simulink model "Pacemaker_AOOR2"  (R2020a)
settings: Solver=FixedStepAuto  StartTime=0.0  StopTime=10.0  FixedStep=1e-3  RelTol=1e-3  EnableMultiTasking=on
libraries: etargetslib x17, frdmk64flib x7, simulink x1
settings Model: ExtModeTrigDuration=5  Creator=Tim_G  LastModifiedBy=Panda
settings OptimizationCC: EnhancedBackFolding=on  PassReuseOutputArgsAs=Individual arguments  ZeroExternalMemoryAtStartup=off  ZeroInternalMemoryAtStartup=off  MaxStackSize=64  OptimizeBlockOrder=speed  DifferentSizesBufferReuse=on  OptimizationCustomize=off  EfficientTunableParamExpr=on
settings DebuggingCC: ParameterTunabilityLossMsg=error
settings HardwareCC: ProdBitPerPointer=32  ProdBitPerSizeT=32  ProdBitPerPtrDiffT=32  ProdLargestAtomicInteger=Long  ProdLargestAtomicFloat=Double  ProdEndianess=BigEndian  ProdWordSize=32  ProdHWDeviceType=ARM Compatible->ARM Cortex
settings SFSimCC: MATLABDynamicMemAlloc=off
settings RTWCC: SystemTargetFile=ert.tlc  HardwareBoard=NXP FRDM-K64F  TemplateMakefile=ert_default_tmf  Toolchain=GNU Tools for ARM Embedded Processors
settings CodeAppCC: ForceParamTrailComments=on  IgnoreCustomStorageClasses=off  OperatorAnnotations=on  SimulinkDataObjDesc=on  SFDataObjDesc=on  InsertBlockDesc=on

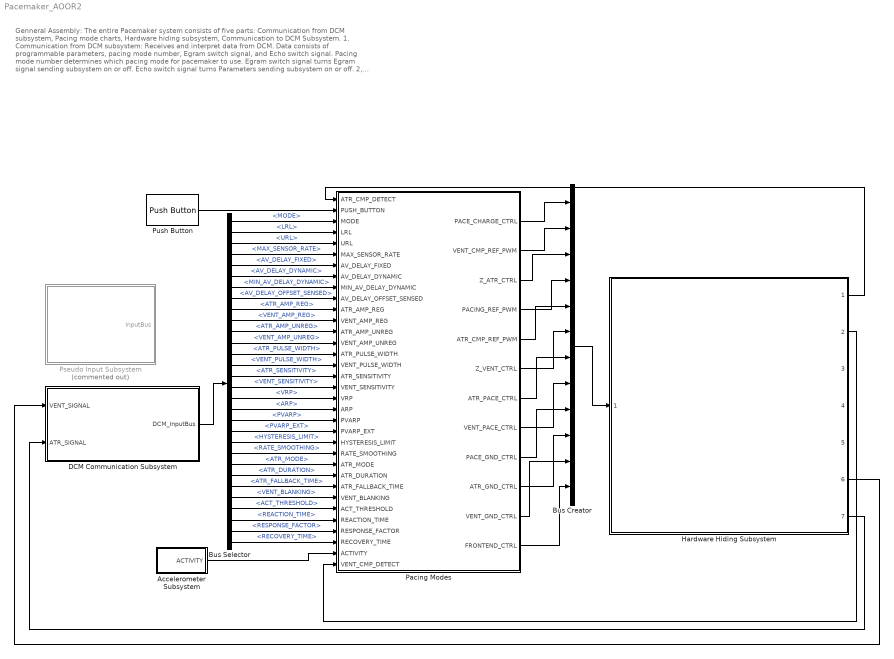
== system Pacemaker_AOOR2 ==
  note: Genneral Assembly:
      |  The entire Pacemaker system consists of five parts: Communication from DCM subsystem, Pacing mode charts, Hardware hiding subsystem, Communication to DCM Subsystem.
      | 1. Communication from DCM subsystem:
      |       Receives and interpret data from DCM. Data consists of programmable parameters, pacing mode number, Egram switch signal, and Echo switch signal.
      |       Pacing mode number determines which pacing mode for pacemaker to use.
      |       Egram switch signal turns Egram signal sending subsystem on or off.
      |       Echo switch signal turns Parameters sending subsystem on or off.
      | 2, Pacing Modes subsystem:
      |       Implementation of different pacing methods. A multiport switch chooses from which pacing mode to output control signals.
      | 3. Hardware hiding subsystem:
      |       Takes control signals as inputs and sends them to the hardware. Also outputs signals received from the hardware.
      | 4. Communication to DCM Subsystem:
      | 	Sends programmable parameters and/or egram signals to DCM if enable signals (ECHO and/or EGRAM) are turned on.
  Accelerometer Subsystem : Subsystem
  Bus Creator : BusCreator  Inputs=12
  Bus Selector : BusSelector  OutputSignals=MODE,LRL,URL,MAX_SENSOR_RATE,AV_DELAY_FIXED,AV_DELAY_DYNAMIC,MIN_AV_DELAY_DYNAMIC,AV_DELAY_OFFSET_SENSED,ATR_AMP_REG,VENT_AMP_REG,ATR_AMP_UNREG,VENT_AMP_UNREG,ATR_PULSE_WIDTH,VENT_PULSE_WIDTH,ATR_SENSITIVITY,VENT_SENSITIVITY,VRP,ARP,PVARP,PVARP_EXT,HYSTERESIS_LIMIT,RATE_SMOOTHING,ATR_MODE,ATR_DURATION,ATR_FALLBACK_TIME,VENT_BLANKING,ACT_THRESHOLD,REACTION_TIME,RESPONSE_FACTOR,RECOVERY_TIME
  DCM Communication Subsystem : Subsystem
  Hardware Hiding Subsystem : Subsystem  ReferencedSubsystem=k64f_hardware_subsystem
  Pacing Modes : Stateflow chart  TreatAsAtomicUnit=on
  Pseudo Input Subsystem : Subsystem  Commented=on
  Push Button : frdmk64flib/Push Button  Whichswitch=SW2  SampleTime1=-1
  wires:
  Hardware Hiding Subsystem/7 -> DCM Communication Subsystem/2(ATR_SIGNAL)
  Hardware Hiding Subsystem/6 -> DCM Communication Subsystem/1(VENT_SIGNAL)
  Push Button/1 -> Pacing Modes/2(PUSH_BUTTON)
  Hardware Hiding Subsystem/1 -> Pacing Modes/1(ATR_CMP_DETECT)
  DCM Communication Subsystem/1(DCM_InputBus) -> Bus Selector/1
  Pacing Modes/1(PACE_CHARGE_CTRL) -> Bus Creator/1
  Pacing Modes/2(VENT_CMP_REF_PWM) -> Bus Creator/2
  Pacing Modes/3(Z_ATR_CTRL) -> Bus Creator/3
  Pacing Modes/4(PACING_REF_PWM) -> Bus Creator/4
  Pacing Modes/5(ATR_CMP_REF_PWM) -> Bus Creator/5
  Pacing Modes/6(Z_VENT_CTRL) -> Bus Creator/6
  Pacing Modes/7(ATR_PACE_CTRL) -> Bus Creator/7
  Pacing Modes/8(VENT_PACE_CTRL) -> Bus Creator/8
  Pacing Modes/9(PACE_GND_CTRL) -> Bus Creator/9
  Pacing Modes/10(ATR_GND_CTRL) -> Bus Creator/10
  Pacing Modes/11(VENT_GND_CTRL) -> Bus Creator/11
  Pacing Modes/12(FRONTEND_CTRL) -> Bus Creator/12
  Bus Creator/1 -> Hardware Hiding Subsystem/1
  Bus Selector/1 -> Pacing Modes/3(MODE)  "<MODE>"
  Bus Selector/2 -> Pacing Modes/4(LRL)  "<LRL>"
  Bus Selector/3 -> Pacing Modes/5(URL)  "<URL>"
  Bus Selector/4 -> Pacing Modes/6(MAX_SENSOR_RATE)  "<MAX_SENSOR_RATE>"
  Bus Selector/5 -> Pacing Modes/7(AV_DELAY_FIXED)  "<AV_DELAY_FIXED>"
  Bus Selector/6 -> Pacing Modes/8(AV_DELAY_DYNAMIC)  "<AV_DELAY_DYNAMIC>"
  Bus Selector/7 -> Pacing Modes/9(MIN_AV_DELAY_DYNAMIC)  "<MIN_AV_DELAY_DYNAMIC>"
  Bus Selector/8 -> Pacing Modes/10(AV_DELAY_OFFSET_SENSED)  "<AV_DELAY_OFFSET_SENSED>"
  Bus Selector/9 -> Pacing Modes/11(ATR_AMP_REG)  "<ATR_AMP_REG>"
  Bus Selector/10 -> Pacing Modes/12(VENT_AMP_REG)  "<VENT_AMP_REG>"
  Bus Selector/11 -> Pacing Modes/13(ATR_AMP_UNREG)  "<ATR_AMP_UNREG>"
  Bus Selector/12 -> Pacing Modes/14(VENT_AMP_UNREG)  "<VENT_AMP_UNREG>"
  Bus Selector/13 -> Pacing Modes/15(ATR_PULSE_WIDTH)  "<ATR_PULSE_WIDTH>"
  Bus Selector/14 -> Pacing Modes/16(VENT_PULSE_WIDTH)  "<VENT_PULSE_WIDTH>"
  Bus Selector/15 -> Pacing Modes/17(ATR_SENSITIVITY)  "<ATR_SENSITIVITY>"
  Bus Selector/16 -> Pacing Modes/18(VENT_SENSITIVITY)  "<VENT_SENSITIVITY>"
  Bus Selector/17 -> Pacing Modes/19(VRP)  "<VRP>"
  Bus Selector/18 -> Pacing Modes/20(ARP)  "<ARP>"
  Bus Selector/19 -> Pacing Modes/21(PVARP)  "<PVARP>"
  Bus Selector/20 -> Pacing Modes/22(PVARP_EXT)  "<PVARP_EXT>"
  Bus Selector/21 -> Pacing Modes/23(HYSTERESIS_LIMIT)  "<HYSTERESIS_LIMIT>"
  Bus Selector/22 -> Pacing Modes/24(RATE_SMOOTHING)  "<RATE_SMOOTHING>"
  Bus Selector/23 -> Pacing Modes/25(ATR_MODE)  "<ATR_MODE>"
  Bus Selector/24 -> Pacing Modes/26(ATR_DURATION)  "<ATR_DURATION>"
  Bus Selector/25 -> Pacing Modes/27(ATR_FALLBACK_TIME)  "<ATR_FALLBACK_TIME>"
  Bus Selector/26 -> Pacing Modes/28(VENT_BLANKING)  "<VENT_BLANKING>"
  Bus Selector/27 -> Pacing Modes/29(ACT_THRESHOLD)  "<ACT_THRESHOLD>"
  Bus Selector/28 -> Pacing Modes/30(REACTION_TIME)  "<REACTION_TIME>"
  Bus Selector/29 -> Pacing Modes/31(RESPONSE_FACTOR)  "<RESPONSE_FACTOR>"
  Bus Selector/30 -> Pacing Modes/32(RECOVERY_TIME)  "<RECOVERY_TIME>"
  Accelerometer Subsystem/1(ACTIVITY) -> Pacing Modes/33(ACTIVITY)
  Hardware Hiding Subsystem/2 -> Pacing Modes/34(VENT_CMP_DETECT)

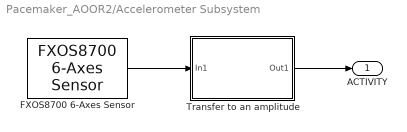
== system Pacemaker_AOOR2/Accelerometer Subsystem ==
  FXOS8700 6-Axes Sensor : frdmk64flib/FXOS8700 6-Axes Sensor  Activesensor=Accelerometer only  ODR=800Hz  HybridODR=400Hz  Accelfullrange=-2g to +2g  SampleTime=-1
  Transfer to an amplitude : Subsystem
  ACTIVITY : Outport
  wires:
  FXOS8700 6-Axes Sensor/1 -> Transfer to an amplitude/1(In1)
  Transfer to an amplitude/1(Out1) -> ACTIVITY/1

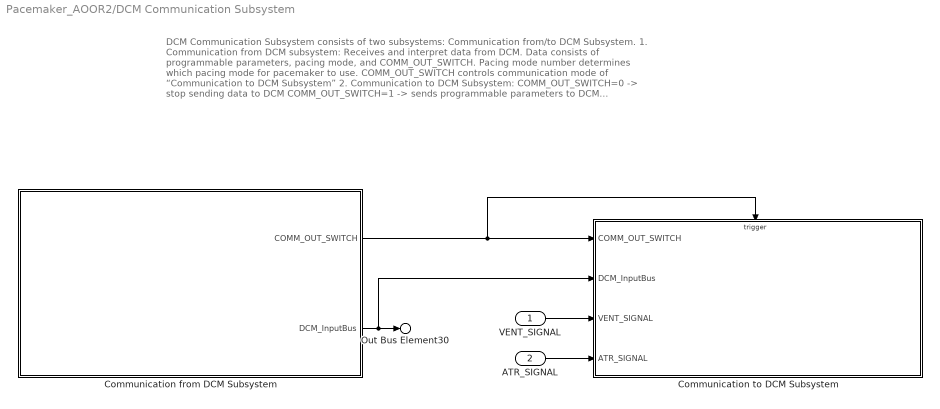
== system Pacemaker_AOOR2/DCM Communication Subsystem ==
  note: DCM Communication Subsystem consists of two subsystems: Communication from/to DCM Subsystem.
      | 1. Communication from DCM subsystem:
      | Receives and interpret data from DCM.
      | Data consists of programmable parameters, pacing mode, and COMM_OUT_SWITCH.
      | Pacing mode number determines which pacing mode for pacemaker to use.
      | COMM_OUT_SWITCH controls communication mode of “Communication to DCM Subsystem”
      | 2. Communication to DCM Subsystem:
      | COMM_OUT_SWITCH=0 -> stop sending data to DCM
      | COMM_OUT_SWITCH=1 -> sends programmable parameters to DCM
      | COMM_OUT_SWITCH=2 -> s ends egram signals to DCM
  VENT_SIGNAL : Inport  OutDataTypeStr=double
  ATR_SIGNAL : Inport  Port=2  OutDataTypeStr=double
  Communication from DCM Subsystem : Subsystem
  Communication to DCM Subsystem : Subsystem  TreatAsAtomicUnit=on
  Out Bus Element30 : Outport  PortName=DCM_InputBus
  wires:
  VENT_SIGNAL/1 -> Communication to DCM Subsystem/3(VENT_SIGNAL)
  ATR_SIGNAL/1 -> Communication to DCM Subsystem/4(ATR_SIGNAL)
  Communication from DCM Subsystem/2(DCM_InputBus) -> Communication to DCM Subsystem/2(DCM_InputBus), Out Bus Element30/1
  Communication from DCM Subsystem/1(COMM_OUT_SWITCH) -> Communication to DCM Subsystem/Trigger, Communication to DCM Subsystem/1(COMM_OUT_SWITCH)

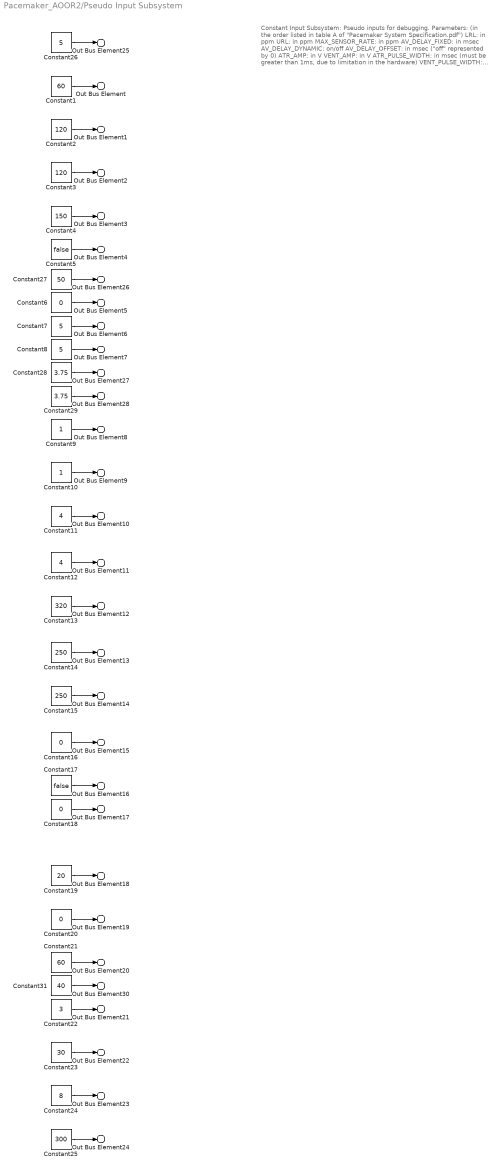
== system Pacemaker_AOOR2/Pseudo Input Subsystem ==
  note: Constant Input Subsystem:
      | Pseudo inputs for debugging.
      |
      | Parameters:
      | (in the order listed in table A of "Pacemaker System Specification.pdf")
      | LRL: in ppm
      | URL: in ppm
      | MAX_SENSOR_RATE: in ppm
      | AV_DELAY_FIXED: in msec
      | AV_DELAY_DYNAMIC: on/off
      | AV_DELAY_OFFSET: in msec ("off" represented by 0)
      | ATR_AMP: in V
      | VENT_AMP: in V
      | ATR_PULSE_WIDTH: in msec (must be greater than 1ms, due to
      | limitation in the hardware)
      | VENT_PULSE_WIDTH: in msec
      | ATR_SENSITIVITY: in V
      | VENT_SENSITIVITY: in V
      | VRP: in msec
      | ARP: in msec
      | PVARP: in msec
      | PVARP_EXT: in msec ("off" represented by 0)
      | HYSTERESIS: off/same choices as LRL (represented by "on")
      | RATE_SMOOTHING: off represented by 0
      | ATR_DURATION: in cardiac cycles
      | ATR_FALLBACK_MODE
      | ATR_FALLBACK_TIME: in sec
      | ACT_THRESHOLD:
      | 0-V-Low
      | 1-Low
      | 2-Med-Low
      | 3-Med
      | 4-Med-High
      | 5-High
      | 6-V-High
      | REACTION_TIME: in sec
      | RESPONSE_FACTOR
      | RECOVERY_TIME: in sec
  Constant1 : Constant  Value=60
  Constant10 : Constant
  Constant11 : Constant  Value=4
  Constant12 : Constant  Value=4
  Constant13 : Constant  Value=320
  Constant14 : Constant  Value=250
  Constant15 : Constant  Value=250
  Constant{6,16,18,20} (4 alike) : Constant  Value=0
  Constant17 : Constant  Value=false
  Constant19 : Constant  Value=20
  Constant2 : Constant  Value=120
  Constant21 : Constant  Value=60
  Constant22 : Constant  Value=3
  Constant23 : Constant  Value=30
  Constant24 : Constant  Value=8
  Constant25 : Constant  Value=300
  Constant26 : Constant  Value=5
  Constant27 : Constant  Value=50
  Constant28 : Constant  Value=3.75
  Constant29 : Constant  Value=3.75
  Constant3 : Constant  Value=120
  Constant31 : Constant  Value=40
  Constant4 : Constant  Value=150
  Constant5 : Constant  Value=false
  Constant7 : Constant  Value=5
  Constant8 : Constant  Value=5
  Constant9 : Constant
  Out Bus Element : Outport  PortName=InputBus  Element=LRL
  Out Bus Element1 : Outport  PortName=InputBus  Element=URL
  Out Bus Element2 : Outport  PortName=InputBus  Element=MAX_SENSOR_RATE
  Out Bus Element3 : Outport  PortName=InputBus  Element=AV_DELAY_FIXED
  Out Bus Element4 : Outport  PortName=InputBus  Element=AV_DELAY_DYNAMIC
  Out Bus Element5 : Outport  PortName=InputBus  Element=AV_DELAY_OFFSET_SENSED
  Out Bus Element6 : Outport  PortName=InputBus  Element=ATR_AMP_REG
  Out Bus Element7 : Outport  PortName=InputBus  Element=VENT_AMP_REG
  Out Bus Element8 : Outport  PortName=InputBus  Element=ATR_PULSE_WIDTH
  Out Bus Element9 : Outport  PortName=InputBus  Element=VENT_PULSE_WIDTH
  Out Bus Element10 : Outport  PortName=InputBus  Element=ATR_SENSITIVITY
  Out Bus Element11 : Outport  PortName=InputBus  Element=VENT_SENSITIVITY
  Out Bus Element12 : Outport  PortName=InputBus  Element=VRP
  Out Bus Element13 : Outport  PortName=InputBus  Element=ARP
  Out Bus Element14 : Outport  PortName=InputBus  Element=PVARP
  Out Bus Element15 : Outport  PortName=InputBus  Element=PVARP_EXT
  Out Bus Element16 : Outport  PortName=InputBus  Element=HYSTERESIS
  Out Bus Element17 : Outport  PortName=InputBus  Element=RATE_SMOOTHING
  Out Bus Element18 : Outport  PortName=InputBus  Element=ATR_DURATION
  Out Bus Element19 : Outport  PortName=InputBus  Element=ATR_FALLBACK_MODE
  Out Bus Element20 : Outport  PortName=InputBus  Element=ATR_FALLBACK_TIME
  Out Bus Element21 : Outport  PortName=InputBus  Element=ACT_THRESHOLD
  Out Bus Element22 : Outport  PortName=InputBus  Element=REACTION_TIME
  Out Bus Element23 : Outport  PortName=InputBus  Element=RESPONSE_FACTOR
  Out Bus Element24 : Outport  PortName=InputBus  Element=RECOVERY_TIME
  Out Bus Element25 : Outport  PortName=InputBus  Element=MODE
  Out Bus Element26 : Outport  PortName=InputBus  Element=MIN_AV_DELAY_DYNAMIC
  Out Bus Element27 : Outport  PortName=InputBus  Element=ATR_AMP_UNREG
  Out Bus Element28 : Outport  PortName=InputBus  Element=VENT_AMP_UNREG
  Out Bus Element30 : Outport  PortName=InputBus  Element=VENT_BLANKING
  wires:
  Constant1/1 -> Out Bus Element/1
  Constant2/1 -> Out Bus Element1/1
  Constant4/1 -> Out Bus Element3/1
  Constant3/1 -> Out Bus Element2/1
  Constant5/1 -> Out Bus Element4/1
  Constant6/1 -> Out Bus Element5/1
  Constant8/1 -> Out Bus Element7/1
  Constant7/1 -> Out Bus Element6/1
  Constant10/1 -> Out Bus Element9/1
  Constant11/1 -> Out Bus Element10/1
  Constant9/1 -> Out Bus Element8/1
  Constant13/1 -> Out Bus Element12/1
  Constant12/1 -> Out Bus Element11/1
  Constant14/1 -> Out Bus Element13/1
  Constant15/1 -> Out Bus Element14/1
  Constant19/1 -> Out Bus Element18/1
  Constant18/1 -> Out Bus Element17/1
  Constant16/1 -> Out Bus Element15/1
  Constant17/1 -> Out Bus Element16/1
  Constant25/1 -> Out Bus Element24/1
  Constant24/1 -> Out Bus Element23/1
  Constant23/1 -> Out Bus Element22/1
  Constant22/1 -> Out Bus Element21/1
  Constant20/1 -> Out Bus Element19/1
  Constant21/1 -> Out Bus Element20/1
  Constant26/1 -> Out Bus Element25/1
  Constant27/1 -> Out Bus Element26/1
  Constant28/1 -> Out Bus Element27/1
  Constant29/1 -> Out Bus Element28/1
  Constant31/1 -> Out Bus Element30/1

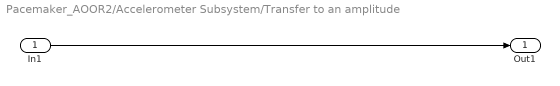
== system Pacemaker_AOOR2/Accelerometer Subsystem/Transfer to an amplitude ==
  In1 : Inport
  Out1 : Outport
  wires:
  In1/1 -> Out1/1

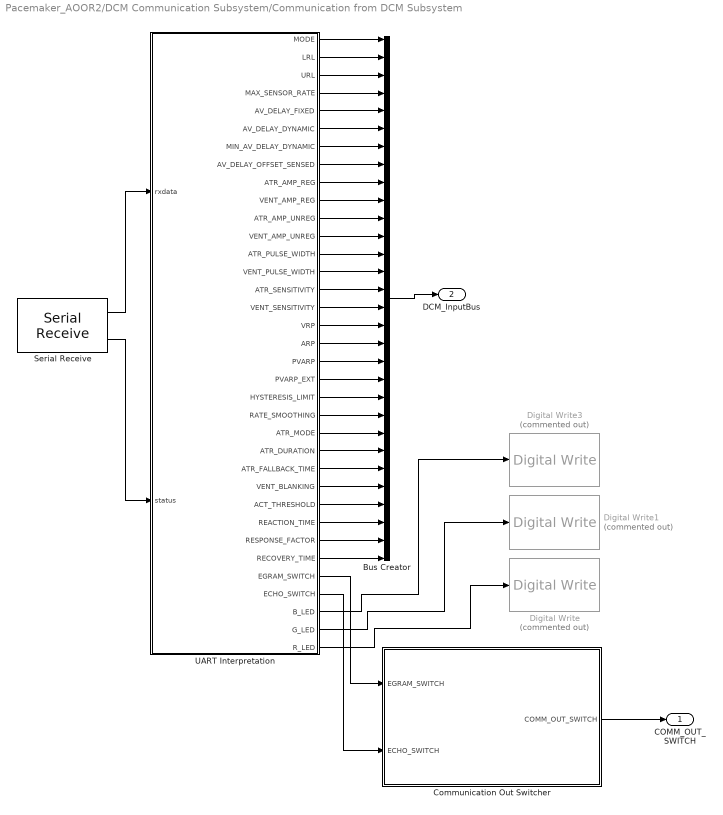
== system Pacemaker_AOOR2/DCM Communication Subsystem/Communication from DCM Subsystem ==
  Bus Creator : BusCreator  Inputs=30
  Communication Out Switcher : Stateflow chart  TreatAsAtomicUnit=on
  Digital Write : frdmk64flib/Digital Write  Commented=on  Whichpin=RED_LED
  Digital Write1 : frdmk64flib/Digital Write  Commented=on  Whichpin=GREEN_LED
  Digital Write3 : frdmk64flib/Digital Write  Commented=on  Whichpin=BLUE_LED
  Serial Receive : frdmk64flib/Serial Receive  SCIModule=0  Baudrate=uint32(9600)  Parity=None  StopBits=1  HardwareFlowControl=None  ByteOrder=LittleEndian  DataType=uint8  DataLength=59  BlockingMode=off  OutputStatus=on  SampleTime=-1
  UART Interpretation : Stateflow chart  TreatAsAtomicUnit=on
  COMM_OUT_SWITCH : Outport
  DCM_InputBus : Outport  Port=2
  wires:
  UART Interpretation/5(AV_DELAY_FIXED) -> Bus Creator/5
  UART Interpretation/14(VENT_PULSE_WIDTH) -> Bus Creator/14
  UART Interpretation/10(VENT_AMP_REG) -> Bus Creator/10
  UART Interpretation/17(VRP) -> Bus Creator/17
  UART Interpretation/6(AV_DELAY_DYNAMIC) -> Bus Creator/6
  UART Interpretation/9(ATR_AMP_REG) -> Bus Creator/9
  UART Interpretation/27(ACT_THRESHOLD) -> Bus Creator/27
  UART Interpretation/24(ATR_DURATION) -> Bus Creator/24
  UART Interpretation/18(ARP) -> Bus Creator/18
  UART Interpretation/8(AV_DELAY_OFFSET_SENSED) -> Bus Creator/8
  UART Interpretation/7(MIN_AV_DELAY_DYNAMIC) -> Bus Creator/7
  Serial Receive/2 -> UART Interpretation/2(status)
  UART Interpretation/3(URL) -> Bus Creator/3
  UART Interpretation/26(VENT_BLANKING) -> Bus Creator/26
  UART Interpretation/13(ATR_PULSE_WIDTH) -> Bus Creator/13
  UART Interpretation/15(ATR_SENSITIVITY) -> Bus Creator/15
  UART Interpretation/11(ATR_AMP_UNREG) -> Bus Creator/11
  UART Interpretation/16(VENT_SENSITIVITY) -> Bus Creator/16
  UART Interpretation/30(RECOVERY_TIME) -> Bus Creator/30
  UART Interpretation/20(PVARP_EXT) -> Bus Creator/20
  UART Interpretation/29(RESPONSE_FACTOR) -> Bus Creator/29
  UART Interpretation/19(PVARP) -> Bus Creator/19
  Serial Receive/1 -> UART Interpretation/1(rxdata)
  UART Interpretation/4(MAX_SENSOR_RATE) -> Bus Creator/4
  UART Interpretation/23(ATR_MODE) -> Bus Creator/23
  UART Interpretation/22(RATE_SMOOTHING) -> Bus Creator/22
  UART Interpretation/12(VENT_AMP_UNREG) -> Bus Creator/12
  UART Interpretation/28(REACTION_TIME) -> Bus Creator/28
  UART Interpretation/25(ATR_FALLBACK_TIME) -> Bus Creator/25
  UART Interpretation/21(HYSTERESIS_LIMIT) -> Bus Creator/21
  UART Interpretation/2(LRL) -> Bus Creator/2
  UART Interpretation/1(MODE) -> Bus Creator/1
  Bus Creator/1 -> DCM_InputBus/1
  Communication Out Switcher/1(COMM_OUT_SWITCH) -> COMM_OUT_SWITCH/1
  UART Interpretation/31(EGRAM_SWITCH) -> Communication Out Switcher/1(EGRAM_SWITCH)
  UART Interpretation/32(ECHO_SWITCH) -> Communication Out Switcher/2(ECHO_SWITCH)
  UART Interpretation/35(R_LED) -> Digital Write/1
  UART Interpretation/33(B_LED) -> Digital Write3/1
  UART Interpretation/34(G_LED) -> Digital Write1/1

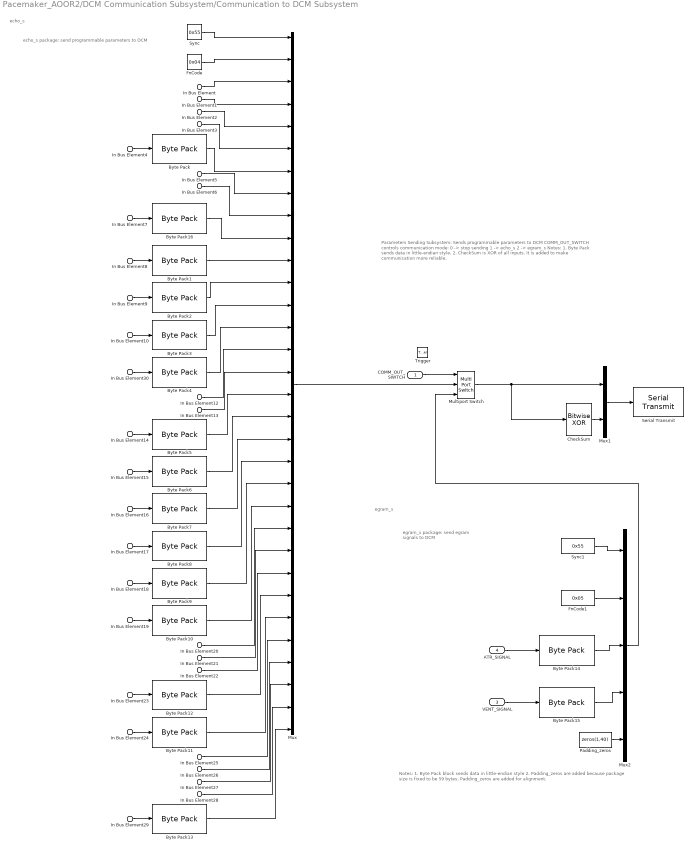
== system Pacemaker_AOOR2/DCM Communication Subsystem/Communication to DCM Subsystem ==
  note: egram_s package:
      | send egram signals to DCM
  note: echo_s package:
      | send programmable parameters to DCM
  note: echo_s
  note: egram_s
  note: Parameters Sending Subsystem:
      | Sends programmable parameters to DCM
      | COMM_OUT_SWITCH controls communication mode:
      | 0 -> stop sending
      | 1 -> echo_s
      | 2 -> egram_s
      | Notes:
      | 1. Byte Pack sends data in little-endian style.
      | 2. CheckSum is XOR of all inputs. It is added to make communication more reliable.
  note: Notes:
      | 1. Byte Pack block sends data in little-endian style
      | 2. Padding_zeros are added because package size is fixed to be 59 bytes. Padding_zeros are added for alignment.
  COMM_OUT_SWITCH : Inport
  In Bus Element : Inport  Port=2  PortName=DCM_InputBus  Element=MODE
  In Bus Element1 : Inport  Port=2  PortName=DCM_InputBus  Element=LRL
  In Bus Element2 : Inport  Port=2  PortName=DCM_InputBus  Element=URL
  In Bus Element3 : Inport  Port=2  PortName=DCM_InputBus  Element=MAX_SENSOR_RATE
  In Bus Element4 : Inport  Port=2  PortName=DCM_InputBus  Element=AV_DELAY_FIXED
  In Bus Element5 : Inport  Port=2  PortName=DCM_InputBus  Element=AV_DELAY_DYNAMIC
  In Bus Element6 : Inport  Port=2  PortName=DCM_InputBus  Element=MIN_AV_DELAY_DYNAMIC
  In Bus Element7 : Inport  Port=2  PortName=DCM_InputBus  Element=AV_DELAY_OFFSET_SENSED
  In Bus Element8 : Inport  Port=2  PortName=DCM_InputBus  Element=ATR_AMP_REG
  In Bus Element9 : Inport  Port=2  PortName=DCM_InputBus  Element=VENT_AMP_REG
  In Bus Element10 : Inport  Port=2  PortName=DCM_InputBus  Element=ATR_AMP_UNREG
  In Bus Element12 : Inport  Port=2  PortName=DCM_InputBus  Element=ATR_PULSE_WIDTH
  In Bus Element13 : Inport  Port=2  PortName=DCM_InputBus  Element=VENT_PULSE_WIDTH
  In Bus Element14 : Inport  Port=2  PortName=DCM_InputBus  Element=ATR_SENSITIVITY
  In Bus Element15 : Inport  Port=2  PortName=DCM_InputBus  Element=VENT_SENSITIVITY
  In Bus Element16 : Inport  Port=2  PortName=DCM_InputBus  Element=VRP
  In Bus Element17 : Inport  Port=2  PortName=DCM_InputBus  Element=ARP
  In Bus Element18 : Inport  Port=2  PortName=DCM_InputBus  Element=PVARP
  In Bus Element19 : Inport  Port=2  PortName=DCM_InputBus  Element=PVARP_EXT
  In Bus Element20 : Inport  Port=2  PortName=DCM_InputBus  Element=HYSTERESIS_LIMIT
  In Bus Element21 : Inport  Port=2  PortName=DCM_InputBus  Element=RATE_SMOOTHING
  In Bus Element22 : Inport  Port=2  PortName=DCM_InputBus  Element=ATR_MODE
  In Bus Element23 : Inport  Port=2  PortName=DCM_InputBus  Element=ATR_DURATION
  In Bus Element24 : Inport  Port=2  PortName=DCM_InputBus  Element=ATR_FALLBACK_TIME
  In Bus Element25 : Inport  Port=2  PortName=DCM_InputBus  Element=VENT_BLANKING
  In Bus Element26 : Inport  Port=2  PortName=DCM_InputBus  Element=ACT_THRESHOLD
  In Bus Element27 : Inport  Port=2  PortName=DCM_InputBus  Element=REACTION_TIME
  In Bus Element28 : Inport  Port=2  PortName=DCM_InputBus  Element=RESPONSE_FACTOR
  In Bus Element29 : Inport  Port=2  PortName=DCM_InputBus  Element=RECOVERY_TIME
  In Bus Element30 : Inport  Port=2  PortName=DCM_InputBus  Element=VENT_AMP_UNREG
  VENT_SIGNAL : Inport  Port=3  OutDataTypeStr=double
  ATR_SIGNAL : Inport  Port=4  OutDataTypeStr=double
  Trigger : TriggerPort  VariantControl=Variant  InitialTriggerSignalState=zero  PortDimensions=1
  Byte Pack{,7..13} (8 alike) : etargetslib/Byte Pack  datatypes={'uint16'}  byteAlign=1
  Byte Pack{1..6} (6 alike) : etargetslib/Byte Pack  datatypes={'single'}  byteAlign=1
  Byte Pack14 : etargetslib/Byte Pack  datatypes={'double'}  byteAlign=1
  Byte Pack15 : etargetslib/Byte Pack  datatypes={'double'}  byteAlign=1
  Byte Pack16 : etargetslib/Byte Pack  datatypes={'int8'}  byteAlign=1
  CheckSum : simulink/Logic and Bit Operations/Bitwise Operator  logicop=XOR  UseBitMask=off  BitMask=bin2dec('11011001')  BitMaskRealWorld=Stored Integer
  FnCode : Constant  Value=0x04  OutDataTypeStr=uint8
  FnCode1 : Constant  Value=0x05  OutDataTypeStr=uint8
  Multiport Switch : MultiPortSwitch  Inputs=2
  Mux : Mux  Inputs=32
  Mux1 : Mux  Inputs=2
  Mux2 : Mux  Inputs=5
  Padding_zeros : Constant  Value=zeros(1,40)  VectorParams1D=off  OutDataTypeStr=uint8
  Serial Transmit : frdmk64flib/Serial Transmit  SCIModule=0  Baudrate=uint32(9600)  Parity=None  StopBits=1  HardwareFlowControl=None  ByteOrder=LittleEndian  BlockingMode=on  OutputStatus=off
  Sync : Constant  Value=0x55  OutDataTypeStr=uint8
  Sync1 : Constant  Value=0x55  OutDataTypeStr=uint8
  wires:
  In Bus Element25/1 -> Mux/28
  Byte Pack13/1 -> Mux/32
  Byte Pack11/1 -> Mux/27
  In Bus Element20/1 -> Mux/23
  Byte Pack12/1 -> Mux/26
  Byte Pack8/1 -> Mux/20
  Byte Pack10/1 -> Mux/22
  In Bus Element/1 -> Mux/3
  Byte Pack9/1 -> Mux/21
  Byte Pack7/1 -> Mux/19
  Byte Pack5/1 -> Mux/17
  In Bus Element12/1 -> Mux/15
  Byte Pack1/1 -> Mux/11
  Byte Pack6/1 -> Mux/18
  In Bus Element6/1 -> Mux/9
  In Bus Element26/1 -> Mux/29
  Byte Pack3/1 -> Mux/13
  Byte Pack2/1 -> Mux/12
  Byte Pack/1 -> Mux/7
  In Bus Element21/1 -> Mux/24
  In Bus Element22/1 -> Mux/25
  In Bus Element28/1 -> Mux/31
  In Bus Element27/1 -> Mux/30
  Byte Pack4/1 -> Mux/14
  In Bus Element13/1 -> Mux/16
  In Bus Element5/1 -> Mux/8
  In Bus Element1/1 -> Mux/4
  In Bus Element4/1 -> Byte Pack/1
  In Bus Element3/1 -> Mux/6
  In Bus Element2/1 -> Mux/5
  FnCode/1 -> Mux/2
  Sync/1 -> Mux/1
  Mux1/1 -> Serial Transmit/1
  CheckSum/1 -> Mux1/2
  Sync1/1 -> Mux2/1
  Mux/1 -> Multiport Switch/2
  Multiport Switch/1 -> CheckSum/1, Mux1/1
  Byte Pack14/1 -> Mux2/3
  Byte Pack15/1 -> Mux2/4
  FnCode1/1 -> Mux2/2
  Mux2/1 -> Multiport Switch/3
  Padding_zeros/1 -> Mux2/5
  Byte Pack16/1 -> Mux/10
  In Bus Element7/1 -> Byte Pack16/1
  In Bus Element8/1 -> Byte Pack1/1
  In Bus Element9/1 -> Byte Pack2/1
  In Bus Element10/1 -> Byte Pack3/1
  In Bus Element30/1 -> Byte Pack4/1
  In Bus Element14/1 -> Byte Pack5/1
  In Bus Element15/1 -> Byte Pack6/1
  In Bus Element16/1 -> Byte Pack7/1
  In Bus Element17/1 -> Byte Pack8/1
  In Bus Element18/1 -> Byte Pack9/1
  In Bus Element19/1 -> Byte Pack10/1
  In Bus Element29/1 -> Byte Pack13/1
  In Bus Element23/1 -> Byte Pack12/1
  In Bus Element24/1 -> Byte Pack11/1
  ATR_SIGNAL/1 -> Byte Pack14/1
  VENT_SIGNAL/1 -> Byte Pack15/1
  COMM_OUT_SWITCH/1 -> Multiport Switch/1

== stateflow chart Pacemaker_AOOR2/DCM Communication Subsystem/Communication from DCM Subsystem/Communication Out Switcher ==
  note: Communication out Switcher:
      | % help switch between echo and egram communication modes
      | 	if ECHO_SWITCH is true:
      | 		send only 1 programmable-parameters package
      | 	If EGRAM_SWITCH is true:
      | 		send a egram data package once per 1ms by switching COMM_OUT_SWITCH between 0/1
  state egram_stop
    % egram low stage
    % wait for 1ms to send next egram package
    entry:
    COMM_OUT_SWITCH=0;
  state comm_stop
    % stop communication
    entry:
    COMM_OUT_SWITCH=0;
  state egram_pulse
    % egram high stage (pulse)
    % send a egram data package
    entry:
    COMM_OUT_SWITCH=2;
  state echo_s_pulse
    % send a programmable-parameters package
    % 1ms delay allows enough time for DCM to read
    entry:
    COMM_OUT_SWITCH=1;
  (default) -> comm_stop
  egram_stop -> comm_stop [order 2] : [ECHO_SWITCH==true]
  comm_stop -> egram_stop [order 2] : [EGRAM_SWITCH==true]
  comm_stop -> (junction 24) [order 1] : [ECHO_SWITCH==true]
  echo_s_pulse -> comm_stop
  egram_pulse -> comm_stop [order 1] : [EGRAM_SWITCH==false | ECHO_SWITCH==true]
  egram_pulse -> egram_stop [order 2]
  egram_stop -> egram_pulse [order 1] : [after(100,msec)]
  (junction 24) -> echo_s_pulse : [after(1,msec)]
  data: EGRAM_SWITCH input boolean; COMM_OUT_SWITCH output uint8; ECHO_SWITCH input boolean

== stateflow chart Pacemaker_AOOR2/DCM Communication Subsystem/Communication from DCM Subsystem/UART Interpretation ==
  settings: executeAtInitialization=1
  state set_r
    entry:
    % store parameters values from DCM
    MODE = data(3);
    LRL = data(4);
    URL = data(5);
    MAX_SENSOR_RATE = data(6);
    AV_DELAY_FIXED = typecast(data(7: 8), 'uint16');
    AV_DELAY_DYNAMIC = data(9);
    MIN_AV_DELAY_DYNAMIC = data(10);
    AV_DELAY_OFFSET_SENSED =  typecast(data(11), 'int8');
    ATR_AMP_REG = typecast(data(12: 15), 'single');
    VENT_AMP_REG = typecast(data(16: 19), 'single');
    ATR_AMP_UNREG = typecast(data(20: 23), 'single');
    VENT_AMP_UNREG = typecast(data(24: 27), 'single');
    ATR_PULSE_WIDTH = data(28);
    VENT_PULSE_WIDTH = data(29);
    ATR_SENSITIVITY = typecast(data(30: 33), 'single');
    VENT_SENSITIVITY = typecast(data(34: 37), 'single');
    VRP = typecast(data(38: 39), 'uint16');
    ARP = typecast(data(40: 41), 'uint16');
    PVARP = typecast(data(42: 43), 'uint16');
    PVARP_EXT = typecast(data(44: 45), 'uint16');
    HYSTERESIS_LIMIT = data(46);
    RATE_SMOOTHING = data(47);
    ATR_MODE = data(48);
    ATR_DURATION = typecast(data(49: 50), 'uint16');
    ATR_FALLBACK_TIME = typecast(data(51: 52), 'uint16');
    VENT_BLANKING = data(53);
    ACT_THRESHOLD = data(54);
    REACTION_TIME = data(55);
    RESPONSE_FACTOR = data(56);
    RECOVERY_TIME = typecast(data(57: 58), 'uint16');
    B_LED=true;
  note: This chart interprets data received from DCM communication.
      | There’re four types of package pacemaker can receive: set_r, echo_r, egram_r, and stopegram_r. (Documentation section 3.3.2)
      | After a package of 59 bytes is received, status==0, then operate the following 4 steps:
      | 1. Validate Sync byte. If not valid, ignore this package and wait for next package.
      | 2. Validate Checksum. If not valid, ignore this package and wait for next package.
      | 3. Operate according to FnCode (set_r, echo_r, egram_r, or stopegram_r).
      | 4. Wait for next package.
      |
      | Note:
      | The matlab function bitsxor() is used to calculate checksum of data received.
  state echo_r
    % send a parameter package to DCM
    entry:
    ECHO_SWITCH=true;
    G_LED=true;
  state Init
    entry:
    % parameters have default values if no data received
    MODE=5; % change to DDD in the future
    LRL=60;
    URL=120;
    MAX_SENSOR_RATE=120;
    AV_DELAY_FIXED=150;
    AV_DELAY_DYNAMIC=0;
    MIN_AV_DELAY_DYNAMIC=50;
    AV_DELAY_OFFSET_SENSED=0;
    ATR_AMP_REG=5;
    VENT_AMP_REG=5;
    ATR_AMP_UNREG=3.75;
    VENT_AMP_UNREG=3.75;
    ATR_PULSE_WIDTH=1;
    VENT_PULSE_WIDTH=1;
    ATR_SENSITIVITY=4;
    VENT_SENSITIVITY=4;
    VRP=320;
    ARP=250;
    PVARP=250;
    PVARP_EXT=0;
    HYSTERESIS_LIMIT=0;
    RATE_SMOOTHING=0;
    ATR_MODE=0;
    ATR_DURATION=20;
    ATR_FALLBACK_TIME=60;
    VENT_BLANKING=40;
    ACT_THRESHOLD=3;
    REACTION_TIME=30;
    RESPONSE_FACTOR=8;
    RECOVERY_TIME=300;
    % local variables that turn egram/echo communication
    % out modules on/off
    EGRAM_SWITCH=false;
    ECHO_SWITCH=false;
  state Checksum
    entry:
    % compare checksum first
    % if checksum is valid, operate according to FnCode
    CHECKSUM=data(59);
    CHECKSUM_REAL=bitsxor(data(1:58));
  state Standby
    %Waiting for Data
    exit:
    % rxdata must be stored initially, otherwise rxdata
    % changes after Checksum. The reason is rxdata
    % reset to zeros after all data have been read
    data=rxdata;
  state stopegram_r
    % stop sending egram to DCM
    entry:
    EGRAM_SWITCH=false;
    R_LED=false;
  state egram_r
    % start sending a egram package
    % to DCM every 1ms
    entry:
    EGRAM_SWITCH=true;
    R_LED=true;
  set_r -> Standby
  (default) -> Init
  (junction 45) -> set_r [order 1] : [data(2)==0x00]
  echo_r -> Standby : {ECHO_SWITCH=false}
  (junction 45) -> Standby [order 5]
  (junction 45) -> echo_r [order 2] : [data(2)==0x01]
  Checksum -> Standby [order 2]
  (junction 41) -> Standby [order 2]
  Checksum -> (junction 45) [order 1] : [CHECKSUM_REAL==CHECKSUM]
  (junction 45) -> egram_r [order 3] : [data(2)==0x02]
  (junction 45) -> stopegram_r [order 4] : [data(2)==0x03]
  Init -> Standby
  Standby -> (junction 41) : [status==0]
  (junction 41) -> Checksum [order 1] : [rxdata(1)==0x55]{B_LED=false;G_LED=false}
  egram_r -> Standby
  stopegram_r -> Standby
  data: checksum function_output uint8 size=1; data_array function_input uint8; MODE output uint8; LRL output uint8; URL output uint8; MAX_SENSOR_RATE output uint8; AV_DELAY_FIXED output uint16; AV_DELAY_DYNAMIC output uint8; MIN_AV_DELAY_DYNAMIC output uint8; AV_DELAY_OFFSET_SENSED output int8; ATR_AMP_REG output single; VENT_AMP_REG output single; ATR_AMP_UNREG output single; VENT_AMP_UNREG output single; ATR_PULSE_WIDTH output uint8; VENT_PULSE_WIDTH output uint8; ATR_SENSITIVITY output single; VENT_SENSITIVITY output single; VRP output uint16; ARP output uint16; PVARP output uint16; PVARP_EXT output uint16; HYSTERESIS_LIMIT output uint8; RATE_SMOOTHING output uint8; ATR_MODE output uint8; ATR_DURATION output uint16; ATR_FALLBACK_TIME output uint16; VENT_BLANKING output uint8; rxdata input uint8; status input uint8; ACT_THRESHOLD output uint8; REACTION_TIME output uint8; RESPONSE_FACTOR output uint8; RECOVERY_TIME output uint16; CHECKSUM_REAL local uint8 size=1; CHECKSUM local uint8 size=1; EGRAM_SWITCH output boolean; ECHO_SWITCH output boolean; B_LED output boolean; data local uint8; G_LED output; R_LED output
  function checksum=bitsxor(data_array):
    | function checksum=bitsxor(data_array)
    |     % calculate checksum
    |     % input: data_array is array of uint8 numbers
    |     % output: checksum (uint8) is bit-wise XOR of all uint8 data in the array
    |     checksum=data_array(1);
    |     for i=2:length(data_array)
    |         checksum = bitxor(checksum,data_array(i)); 
    |     end
    | end

== stateflow chart Pacemaker_AOOR2/Pacing Modes ==
  state Pacing_Modes_Switch
    % switch pacing modes according to MODE
    % similar to switch case in C = C + 1
  state AOO
    note: AOO Pacing Mode:
        |
        | Inputs:
        | ppm=LRL; (1/automatic interval)
        | ATR_AMP_REG; (amplitude in V)
        | ATR_PULSE_WIDTH; (in msec)
    state Init
      entry:
      VENT_CMP_REF_PWM=100;
      ATR_CMP_REF_PWM=100;
      FRONTEND_CTRL=false;
    state Charging
      %% Charge C22
      entry:
      ATR_PACE_CTRL = false;
      VENT_PACE_CTRL = false;
      PACING_REF_PWM = double(ATR_AMP_REG*20);
      % Because 0-100% PWM corresponds to 0-5V output,
      % PWM duty cycle = ATR_AMP_REG/5*100;
      PACE_CHARGE_CTRL = true;
      %% Discharge C21
      PACE_GND_CTRL = true;
      Z_ATR_CTRL = false;
      Z_VENT_CTRL = false;
      ATR_GND_CTRL = true;
      VENT_GND_CTRL = false;
    state Pacing
      entry:
      PACE_CHARGE_CTRL = false;
      PACE_GND_CTRL = true;
      ATR_PACE_CTRL = true;
      ATR_GND_CTRL = false;
      Z_ATR_CTRL = false;
      Z_VENT_CTRL =false;
      VENT_GND_CTRL = false;
      VENT_PACE_CTRL = false;
    (default) -> AOO.Init
    AOO.Charging -> AOO.Pacing : [after(60/LRL,sec)]
    AOO.Init -> AOO.Charging
    AOO.Pacing -> AOO.Charging : [after(ATR_PULSE_WIDTH,msec)]
  state VOO [commented out]
    note: VOO Pacing Mode:
        |
        | Inputs:
        | ppm=LRL; (1/automatic interval)
        | VENT_AMP_REG; (amplitude in V)
        | VENT_PULSE_WIDTH; (in msec)
    state Init [commented out]
      entry:
      VENT_CMP_REF_PWM=100;
      ATR_CMP_REF_PWM=100;
      FRONTEND_CTRL=false;
    state Charging [commented out]
      entry:
      %% Charge C22
      ATR_PACE_CTRL = false;
      VENT_PACE_CTRL = false;
      PACING_REF_PWM = double(VENT_AMP_REG*20);
      % Because 0-100% PWM corresponds to 0-5V output,
      %PWM duty cycle = VENT_AMP_REG/5*100;
      PACE_CHARGE_CTRL = true;
      %% Discharge C21
      PACE_GND_CTRL = true;
      Z_ATR_CTRL = false;
      Z_VENT_CTRL = false;
      ATR_GND_CTRL = false;
      VENT_GND_CTRL = true;
    state Pacing [commented out]
      entry:
      PACE_CHARGE_CTRL = false;
      PACE_GND_CTRL = true;
      ATR_PACE_CTRL = false;
      ATR_GND_CTRL = false;
      Z_ATR_CTRL = false;
      Z_VENT_CTRL = false;
      VENT_GND_CTRL = false;
      VENT_PACE_CTRL = true;
    (default) -> VOO.Init [commented out]
    VOO.Charging -> VOO.Pacing [commented out] : [after(60/LRL,sec)]
    VOO.Pacing -> VOO.Charging [commented out] : [after(VENT_PULSE_WIDTH,msec)]
    VOO.Init -> VOO.Charging [commented out]
  state AAI [commented out]
    state REF_delay [commented out]
    note: Inputs:
        | ATR_SENSITIVITY (sensing threshold in V)
        | ARP; (atrial refactory period, in msec)
        | ppm= LRL; (1/automatic interval)
        | ATR_AMP_REG (amplitude in V)
        | ATR_PULSE_WIDTH; (pulse width in msec)
        | ATR_CMP_DETECT; (sensing signal from hardware)
    state Sensing [commented out]
      entry:
      FRONTEND_CTRL = true;
      VENT_CMP_REF_PWM=100;
      ATR_CMP_REF_PWM = double(ATR_SENSITIVITY*20);
      % see explanation for ...REF_PWM in section 2.3.4 of the Document
    state Charge [commented out]
      entry:
      %% Charge C22
      ATR_PACE_CTRL = false;
      VENT_PACE_CTRL = false;
      PACING_REF_PWM = double(ATR_AMP_REG*20);
      % Because 0-100% PWM corresponds to 0-5V output,
      % PWM duty cycle = ATR_AMP_REG/5*100;
      PACE_CHARGE_CTRL = true;
      %% Discharge C21
      PACE_GND_CTRL = true;
      Z_ATR_CTRL = false;
      Z_VENT_CTRL = false;
      ATR_GND_CTRL = true;
      VENT_GND_CTRL = false;
    state Pacing [commented out]
      entry:
      PACE_CHARGE_CTRL = false;
      PACE_GND_CTRL = true;
      ATR_PACE_CTRL = true;
      ATR_GND_CTRL = false;
      Z_ATR_CTRL = false;
      Z_VENT_CTRL = false;
      VENT_GND_CTRL = false;
      VENT_PACE_CTRL = false;
    AAI.REF_delay -> AAI.Pacing [commented out] : [after(60000/LRL - double(ATR_PULSE_WIDTH) - double(ARP), msec)]
    Charge -> AAI.REF_delay [commented out] : [after(ARP,msec)]
    AAI.REF_delay -> Charge [commented out] : [ATR_CMP_DETECT == true || PUSH_BUTTON==true]
    (default) -> Sensing [commented out]
    Sensing -> Charge [commented out]
    AAI.Pacing -> Charge [commented out] : [after(ATR_PULSE_WIDTH,msec)]
  state VVI [commented out]
    state REF_delay [commented out]
    note: Inputs
        | VENT_SENSITIVITY; (sensing threshold in V)
        | VRP; (ventricular refactory period, in msec)
        | ppm=LRL; (1/automatic interval)
        | VENT_AMP; (amplitude in V)
        | VENT_PULSE_WIDTH; (in msec)
        | VENT_CMP_DETECT (sensing signal from hardware)
    state Init [commented out]
      entry:
      FRONTEND_CTRL = true;
      ATR_CMP_REF_PWM=100;
      VENT_CMP_REF_PWM =double(VENT_SENSITIVITY*20);
      % see explanation for ...REF_PWM in section 2.3.4 of the Document
    state Charging [commented out]
      entry:
      %% Charge C22
      ATR_PACE_CTRL = false;
      VENT_PACE_CTRL = false;
      PACING_REF_PWM = double(VENT_AMP_REG*20);
      % Because 0-100% PWM corresponds to 0-5V output,
      % PWM duty cycle = VENT_AMP_REG/5*100;
      PACE_CHARGE_CTRL = true;
      %% Discharge C21
      PACE_GND_CTRL = true;
      Z_ATR_CTRL = false;
      Z_VENT_CTRL = false;
      ATR_GND_CTRL = false;
      VENT_GND_CTRL = true;
    state Pacing [commented out]
      entry:
      PACE_CHARGE_CTRL = false;
      PACE_GND_CTRL = true;
      ATR_PACE_CTRL = false;
      ATR_GND_CTRL = false;
      Z_ATR_CTRL = false;
      Z_VENT_CTRL = false;
      VENT_GND_CTRL = false;
      VENT_PACE_CTRL = true;
    VVI.REF_delay -> VVI.Pacing [commented out] : [after(60000/LRL - double(VENT_PULSE_WIDTH) - double(VRP), msec)]
    VVI.Charging -> VVI.REF_delay [commented out] : [after(VRP,msec)]
    VVI.REF_delay -> VVI.Charging [commented out] : [VENT_CMP_DETECT == true || PUSH_BUTTON==true]
    (default) -> VVI.Init [commented out]
    VVI.Pacing -> VVI.Charging [commented out] : [after(VENT_PULSE_WIDTH,msec)]
    VVI.Init -> VVI.Charging [commented out]
  state AOOR [commented out]
    state Very_High_Threshold [commented out]
      entry:
      ACTIVITY_THRESHOLD=2;
    state High_Threshold [commented out]
      entry:
      ACTIVITY_THRESHOLD=1.75;
    state Pacing [commented out]
      entry:
      PACE_CHARGE_CTRL = false;
      PACE_GND_CTRL = true;
      ATR_PACE_CTRL = true;
      ATR_GND_CTRL = false;
      Z_ATR_CTRL = false;
      Z_VENT_CTRL =false;
      VENT_GND_CTRL = false;
      VENT_PACE_CTRL = false;
    state Medium_High_Threshold [commented out]
      entry:
      ACTIVITY_THRESHOLD=1.4;
    state AOOR_Charge [commented out]
      state CHARGE [commented out]
        entry:
        %% Charge C22
        entry:
        ATR_PACE_CTRL = false;
        VENT_PACE_CTRL = false;
        PACING_REF_PWM = double(ATR_AMP_REG*20);
        % Because 0-100% PWM corresponds to 0-5V output,
        % PWM duty cycle = ATR_AMP_REG/5*100;
        PACE_CHARGE_CTRL = true;
        %% Discharge C21
        PACE_GND_CTRL = true;
        Z_ATR_CTRL = false;
        Z_VENT_CTRL = false;
        ATR_GND_CTRL = true;
        VENT_GND_CTRL = false;
        %%get the vector norm of activity
        ACTIVITY_NORM = sqrt(ACTIVITY(1)^2+ACTIVITY(2)^2+ACTIVITY(3)^2);
      state More_than_threshold [commented out]
        entry:
        TARGET = (MAX_SENSOR_RATE - LRL) * (RESPONSE_FACTOR / 16) + LRL;
      state Less_than_threshold [commented out]
        entry:
        TARGET = LRL;
      state Increse_HR [commented out]
        entry:
        % Reaction time is in seconds
        SLOPE=(MAX_SENSOR_RATE - LRL)/REACTION_TIME;
        % step is increase in LRL_TARGET after 60/LRL_TARGET time
        STEP = SLOPE*(60/LRL_TARGET);
        LRL_TARGET = LRL_TARGET + STEP;
        B_LED=true;
        R_LED=false;
        G_LED=false;
      state Decrese_HR [commented out]
        entry:
        % Recovery time is in seconds
        SLOPE=(MAX_SENSOR_RATE-LRL)/RECOVERY_TIME;
        STEP = SLOPE*(60/LRL_TARGET);
        LRL_TARGET = LRL_TARGET - STEP;
        G_LED=true;
        R_LED=false;
        B_LED=false;
      state Maintain_HR [commented out]
        % no change to LRL_TARGET
        %%B_LED=true;
        entry:
        R_LED=true;
        G_LED=false;
        B_LED=false;
      (default) -> CHARGE [commented out]
      CHARGE -> More_than_threshold [commented out] : [ACTIVITY_NORM >= ACTIVITY_THRESHOLD]
      CHARGE -> Less_than_threshold [commented out] : [ACTIVITY_NORM< ACTIVITY_THRESHOLD]
      Less_than_threshold -> Maintain_HR [commented out] : [PREV_LRL <= TARGET]
      More_than_threshold -> Increse_HR [commented out] : [LRL_TARGET < TARGET]
      More_than_threshold -> Maintain_HR [commented out] : [PREV_LRL >= TARGET]
      Less_than_threshold -> Decrese_HR [commented out] : [LRL_TARGET > TARGET]
    state Init [commented out]
      entry:
      ATR_CMP_REF_PWM=100;
      VENT_CMP_REF_PWM=100;
      FRONTEND_CTRL=false;
      LRL_TARGET = LRL;
    state Medium_Threshold [commented out]
      % if no match value for ACT_THRESHOLD, use medium as default
      entry:
      ACTIVITY_THRESHOLD=1.15;
    state Medium_Low_Threshold [commented out]
      entry:
      ACTIVITY_THRESHOLD=1.1;
    state Low_Threshold [commented out]
      entry:
      ACTIVITY_THRESHOLD=1.05;
    state Very_Low_Threshold [commented out]
      entry:
      ACTIVITY_THRESHOLD=1.01;
    Very_High_Threshold -> AOOR_Charge [commented out]
    (junction 180) -> Very_High_Threshold [commented out] : [ACT_THRESHOLD==6]
    High_Threshold -> AOOR_Charge [commented out]
    (junction 180) -> High_Threshold [commented out] : [ACT_THRESHOLD==5]
    (default) -> AOOR.Init [commented out]
    Medium_High_Threshold -> AOOR_Charge [commented out]
    (junction 180) -> Medium_High_Threshold [commented out] : [ACT_THRESHOLD==4]
    AOOR.Pacing -> AOOR_Charge [commented out] : [after(ATR_PULSE_WIDTH,msec)]
    Medium_Threshold -> AOOR_Charge [commented out]
    AOOR.Init -> (junction 180) [commented out]
    (junction 180) -> Medium_Threshold [commented out]
    (junction 180) -> Medium_Low_Threshold [commented out] : [ACT_THRESHOLD==2]
    (junction 180) -> Low_Threshold [commented out] : [ACT_THRESHOLD==1]
    (junction 180) -> Very_Low_Threshold [commented out] : [ACT_THRESHOLD==0]
    AOOR_Charge -> AOOR.Pacing [commented out] : [after(60000/LRL_TARGET-ATR_PULSE_WIDTH,msec)]
    Very_Low_Threshold -> AOOR_Charge [commented out]
    Medium_Low_Threshold -> AOOR_Charge [commented out]
    Low_Threshold -> AOOR_Charge [commented out]
  (default) -> Pacing_Modes_Switch
  Pacing_Modes_Switch -> AOO : [MODE==5]
  AOO -> Pacing_Modes_Switch : [MODE~=5]
  Pacing_Modes_Switch -> VOO [commented out] : [MODE==7]
  VOO -> Pacing_Modes_Switch [commented out] : [MODE~=7]
  Pacing_Modes_Switch -> AAI [commented out] : [MODE==6]
  AAI -> Pacing_Modes_Switch [commented out] : [MODE~=6]
  Pacing_Modes_Switch -> VVI [commented out] : [MODE==8]
  VVI -> Pacing_Modes_Switch [commented out] : [MODE~=8]
  Pacing_Modes_Switch -> AOOR [commented out] : [MODE==15]
  AOOR -> Pacing_Modes_Switch [commented out] : [MODE~=15]
  data: ATR_CMP_DETECT input boolean size=1; PACE_CHARGE_CTRL output boolean; VENT_CMP_REF_PWM output double; Z_ATR_CTRL output boolean; PUSH_BUTTON input boolean; PACING_REF_PWM output double; ATR_CMP_REF_PWM output double; Z_VENT_CTRL output boolean; ATR_PACE_CTRL output boolean; VENT_PACE_CTRL output boolean; PACE_GND_CTRL output boolean; ATR_GND_CTRL output boolean; VENT_GND_CTRL output boolean; FRONTEND_CTRL output boolean; MODE input uint8; LRL input uint8; URL input uint8; MAX_SENSOR_RATE input uint8; AV_DELAY_FIXED input uint16; AV_DELAY_DYNAMIC input uint8; MIN_AV_DELAY_DYNAMIC input uint8; AV_DELAY_OFFSET_SENSED input int8; ATR_AMP_REG input single; VENT_AMP_REG input single; ATR_AMP_UNREG input single; VENT_AMP_UNREG input single; ATR_PULSE_WIDTH input uint8; VENT_PULSE_WIDTH input uint8; ATR_SENSITIVITY input single; VENT_SENSITIVITY input single; VRP input uint16; ARP input uint16; PVARP input uint16; PVARP_EXT input uint16; HYSTERESIS_LIMIT input uint8; RATE_SMOOTHING input uint8; ATR_MODE input uint8; ATR_DURATION input uint16; ATR_FALLBACK_TIME input uint16; VENT_BLANKING input uint8; ACT_THRESHOLD input uint8; REACTION_TIME input uint8; RESPONSE_FACTOR input uint8; RECOVERY_TIME input uint16; ACTIVITY input; ACTIVITY_NORM local; LRL_TARGET local; SLOPE local; STEP local; TARGET local; VENT_CMP_DETECT input boolean size=1; ACTIVITY_THRESHOLD local double
